simulink model "Gradient_Descent_Sleep_Advance"  (R2015a)
settings: Solver=ode5  StartTime=0.0  StopTime=350  FixedStep=0.01  MaxStep=0.01  RelTol=1e-3
values from neighbouring files (symbols this model uses):
  H0 = interp1q(Periodic_Solution(:,1),Periodic_Solution(:,3),Initial_Time-6)    [Gradient_Descent_Controllable_Sleeping.m]
  Periodic_Solution = Periodic_Solution(N:end,:)    [Gradient_Descent_Controllable_Sleeping.m]    (also in Periodic_Solution_PRC_u_1000lux.mat = [0 0.00999999999999 0.02 0.03 0.04 0.05 0.0599999999999 0.06)
  Sleep = sleep    [Gradient_Descent_Controllable_Sleeping.m]
  Sleep0 = 0    [Gradient_Descent_Controllable_Sleeping.m]
  theta0 = interp1q(Periodic_Solution(:,1),Periodic_Solution(:,2),Initial_Time-6)    [Gradient_Descent_Controllable_Sleeping.m]
  tol = 0.01    [Gradient_Descent_Controllable_Sleeping.m]
  umax = 0.2208    [Gradient_Descent_Controllable_Sleeping.m]
undefined symbols (not defined in the file or in its folder): f
settings Model: Creator=wangf7  LastModifiedBy=Jiawei Yin
settings OptimizationCC: ExpressionDepthLimit=2147483647
settings DebuggingCC: AlgebraicLoopMsg=none  ArtificialAlgebraicLoopMsg=none  UnderspecifiedInitializationDetection=Classic  MergeDetectMultiDrivingBlocksExec=none  SolverPrmCheckMsg=warning  StateNameClashWarn=warning

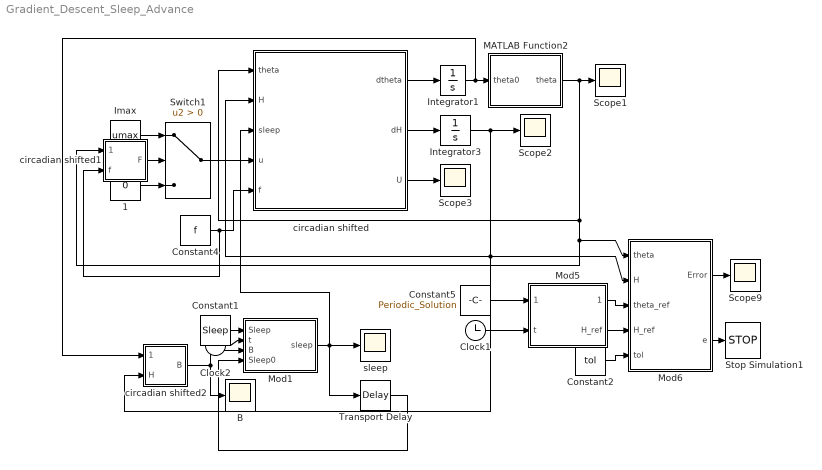
== system Gradient_Descent_Sleep_Advance ==
  1 : Constant  Value=0
  B : Scope
      settings: TimeRange=auto  MaxDataPoints=5000000000  SaveName=B  YMin=0.1808  YMax=0.82676  SampleTime=-1  DataFormat=Array
  Clock1 : Clock
  Clock2 : Clock
  Constant1 : Constant  Value=Sleep
  Constant2 : Constant  Value=tol
  Constant4 : Constant  Value=f
  Constant5 : Constant  Value=Periodic_Solution
  Imax : Constant  Value=umax
  Integrator1 : Integrator  InitialCondition=theta0
  Integrator3 : Integrator  InitialCondition=H0
  MATLAB Function2 : MATLAB Function  TreatAsAtomicUnit=on
      settings: PermitHierarchicalResolution=ParametersOnly
  Mod1 : MATLAB Function  TreatAsAtomicUnit=on
      settings: PermitHierarchicalResolution=ParametersOnly
  Mod5 : MATLAB Function  TreatAsAtomicUnit=on
      settings: PermitHierarchicalResolution=ParametersOnly
  Mod6 : MATLAB Function  TreatAsAtomicUnit=on
      settings: PermitHierarchicalResolution=ParametersOnly
  Scope{1..3,9} (4 alike) : Scope
      Scope1 settings: TimeRange=auto  MaxDataPoints=5000000000  SaveName=theta  YMin=-0.78504  YMax=7.06814  SampleTime=-1  DataFormat=Array
      Scope2 settings: TimeRange=auto  MaxDataPoints=5000000000  SaveName=H  YMin=0.15315  YMax=0.16049  SampleTime=-1  DataFormat=Array
      Scope3 settings: TimeRange=auto  MaxDataPoints=5000000000  SaveName=u  YMin=-0.0299  YMax=0.2691  SampleTime=-1  DataFormat=Array
      Scope9 settings: TimeRange=auto  MaxDataPoints=5000000000  SaveName=Error  YMin=-0.08503  YMax=0.86612  SampleTime=-1  DataFormat=Array
  Stop Simulation1 : Stop
  Switch1 : Switch  Criteria=u2 > Threshold
  Transport Delay : TransportDelay  DelayTime=.01  InitialOutput=Sleep0
  circadian shifted : MATLAB Function  TreatAsAtomicUnit=on
      settings: PermitHierarchicalResolution=ParametersOnly
  circadian shifted1 : MATLAB Function  TreatAsAtomicUnit=on
      settings: PermitHierarchicalResolution=ParametersOnly
  circadian shifted2 : MATLAB Function  TreatAsAtomicUnit=on
      settings: PermitHierarchicalResolution=ParametersOnly
  sleep : Scope
      settings: TimeRange=auto  MaxDataPoints=5000000000  SaveName=sleep  YMin=-0.125  YMax=1.125  SampleTime=-1  DataFormat=Array
  wires:
  Imax/1 -> Switch1/1
  1/1 -> Switch1/3
  Switch1/1 -> circadian shifted/4(u)
  Constant4/1 -> circadian shifted1/2(f), circadian shifted/5(f)
  circadian shifted/1(dtheta) -> Integrator1/1
  circadian shifted/2(dH) -> Integrator3/1
  Integrator1/1 -> circadian shifted2/1(theta), MATLAB Function2/1(theta0)
  MATLAB Function2/1(theta) -> circadian shifted1/1(theta), Mod6/1(theta), circadian shifted/1(theta), Scope1/1
  Integrator3/1 -> circadian shifted2/2(H), Mod6/2(H), circadian shifted/2(H), Scope2/1
  Constant5/1 -> Mod5/1(Periodic_Solution)
  Clock1/1 -> Mod5/2(t)
  Mod6/2(e) -> Stop Simulation1/1
  Mod6/1(Error) -> Scope9/1
  Mod5/1(theta_ref) -> Mod6/3(theta_ref)
  Mod5/2(H_ref) -> Mod6/4(H_ref)
  circadian shifted1/1(F) -> Switch1/2
  Constant2/1 -> Mod6/5(tol)
  circadian shifted/3(U) -> Scope3/1
  Constant1/1 -> Mod1/1(Sleep)
  Clock2/1 -> Mod1/2(t)
  Mod1/1(sleep) -> Transport Delay/1, sleep/1, circadian shifted/3(sleep)
  circadian shifted2/1(B) -> Mod1/3(B), B/1
  Transport Delay/1 -> Mod1/4(Sleep0)

== matlab function Gradient_Descent_Sleep_Advance/circadian shifted1 ==
  data: theta input; f input; F output
function F = fcn(theta,f)
%#eml
F=interp1q(f(:,1),f(:,2),theta);

== matlab function Gradient_Descent_Sleep_Advance/Mod1 ==
  data: Sleep input; sleep output; t input; B input; Sleep0 input
function sleep = fcn(Sleep,t,B,Sleep0)
%#codegen
if t<=Sleep(end,1)
    sleep=interp1q(Sleep(:,1),Sleep(:,2),t);
    if round(sleep)==0 && round(Sleep0)==1
        if B>0.27
            sleep=1;
        end
    elseif round(sleep)==1 && round(Sleep0)==0
        if B<0.67
            sleep=0;
        end
    end
    if B>=0.77
        sleep=1;
    elseif B<=0.17
        sleep=0;
    end
else
    sleep=round(Sleep0);
    if B>=0.67
        sleep=1;
    elseif B<=0.17
        sleep=0;
    end
end

== matlab function Gradient_Descent_Sleep_Advance/circadian shifted2 ==
  data: theta input; H input; B output
function B = fcn(theta,H)
%#eml
B=H-0.1333*cos(theta);

== matlab function Gradient_Descent_Sleep_Advance/circadian shifted ==
  data: theta input; H input; sleep input; u input; dtheta output; dH output; f input; U output
function [dtheta,dH,U] = fcn(theta,H,sleep,u,f)
%#eml
omega0=2*pi/24.2;
tr=18.2;
td=4.2;
U=(1-sleep)*u;
if sleep==0
    dtheta=omega0+interp1q(f(:,1),f(:,2),theta)*u;
    dH=(1-H)/tr;
else
    dtheta=omega0;
    dH=-H/td;
end

== matlab function Gradient_Descent_Sleep_Advance/MATLAB Function2 ==
  data: theta0 input; theta output
function theta  = fcn(theta0)

theta=mod(theta0,2*pi);

== matlab function Gradient_Descent_Sleep_Advance/Mod5 ==
  data: Periodic_Solution input; theta_ref output; t input; H_ref output
function [theta_ref,H_ref] = fcn(Periodic_Solution,t)
%#codegen
theta_ref=interp1q(Periodic_Solution(:,1),Periodic_Solution(:,2),t);
H_ref=interp1q(Periodic_Solution(:,1),Periodic_Solution(:,3),t);

== matlab function Gradient_Descent_Sleep_Advance/Mod6 ==
  data: Error output; theta input; H input; e output; theta_ref input; H_ref input; tol input
function [Error,e] = fcn(theta,H,theta_ref,H_ref,tol)
%#codegen
Error=(H-H_ref)^2+min([(theta-theta_ref)^2,(theta-theta_ref-2*pi)^2,(theta-theta_ref+2*pi)^2]);
e=Error<tol;
